simulink model "Heating_system"  (R2021a)
settings: Solver=VariableStepAuto  StartTime=0.0  StopTime=inf  RelTol=1e-3
settings Model: DataDictionary=Thermostat.sldd  EnablePacing=on  PacingRate=0.350000  OrderedModelArguments=off  Creator=smrh1  LastModifiedBy=smrh1

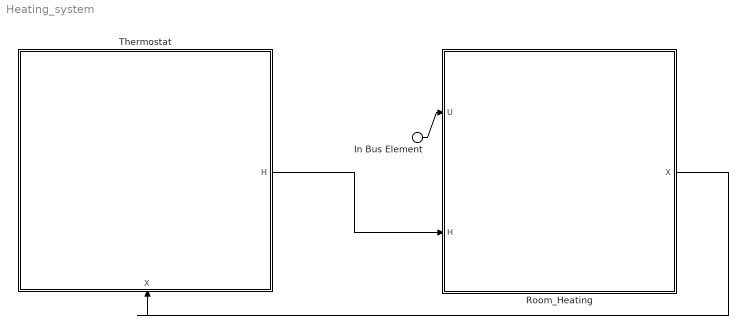
== system Heating_system ==
  In Bus Element : Inport  PortName=U
  Room_Heating : Subsystem
      settings: PortSchema="{\"entries\":[{\"content\":{\"headerSize\":26,\"margin\":15,\"minimumSpacing\":25,\"sides\":[{\"content\":{\"connectorIds\":[\"In1\",\"In2\"]},\"type\":\"ConnectorPlacement.EquallySpacedRectSide\",\"uuid\":\"3399fd0f-e173-41a6-b187-8436c8bfa551\"},{\"content\":{\"connectorIds\":[\"Out1\"],\"side\":\"RIGHT\"},\"type\":\"ConnectorPlacement.EquallySpacedRectSide\",\"uuid\":\"ade3010a-e700-4d19-9692-9b4fbd9f77bd\"},{\"content\":{\"connectorIds\":[],\"side\":\"TOP\"},\"type\":\"ConnectorPlacement.EquallySpacedRectSide\",\"uuid\":\"996f7f95-9ab9-4e94-926a-d72fb20bb1ec\"}]},\"type\":\"ConnectorPlacement.EquallySpacedConnector\",\"uuid\":\"0c58a4e7-12d7-4b31-b33f-6c78252624a7\"}],\"packageUris\":[\"http://schema.mathworks.com/mf0/Connector/R2020b\"],\"version\":\"1.0\"}"
  Thermostat : Subsystem
      settings: PortSchema="{\"entries\":[{\"content\":{\"headerSize\":26,\"margin\":15,\"minimumSpacing\":25,\"sides\":[{\"content\":{\"connectorIds\":[]},\"type\":\"ConnectorPlacement.EquallySpacedRectSide\",\"uuid\":\"3399fd0f-e173-41a6-b187-8436c8bfa551\"},{\"content\":{\"connectorIds\":[\"Out1\"],\"side\":\"RIGHT\"},\"type\":\"ConnectorPlacement.EquallySpacedRectSide\",\"uuid\":\"ade3010a-e700-4d19-9692-9b4fbd9f77bd\"},{\"content\":{\"connectorIds\":[],\"side\":\"TOP\"},\"type\":\"ConnectorPlacement.EquallySpacedRectSide\",\"uuid\":\"996f7f95-9ab9-4e94-926a-d72fb20bb1ec\"},{\"content\":{\"connectorIds\":[\"In1\"],\"side\":\"BOTTOM\"},\"type\":\"ConnectorPlacement.EquallySpacedRectSide\",\"uuid\":\"850434b0-8785-4975-a631-b4ec0ca1fe29\"}]},\"type\":\"ConnectorPlacement.EquallySpacedConnector\",\"uuid\":\"0c58a4e7-12d7-4b31-b33f-6c78252624a7\"}],\"packageUris\":[\"http://schema.mathworks.com/mf0/Connector/R2020b\"],\"version\":\"1.0\"}"
  wires:
  Thermostat/1(H) -> Room_Heating/2(H)
  In Bus Element/1 -> Room_Heating/1(U)
  Room_Heating/1(X) -> Thermostat/1(X)

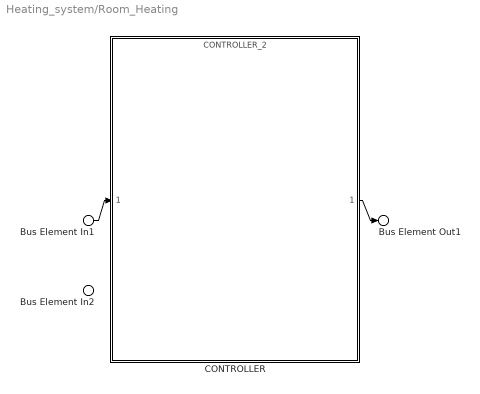
== system Heating_system/Room_Heating ==
  Bus Element In2 : Inport  PortName=U
  Bus Element In1 : Inport  Port=2  PortName=H
  CONTROLLER : ModelReference  ModelNameDialog=CONTROLLER_2  SimulationMode=Normal  ModelReferenceVersion=1.8
      settings: PortSchema="{\"entries\":[{\"content\":{\"headerSize\":38,\"margin\":15,\"minimumSpacing\":25,\"sides\":[{\"content\":{\"connectorIds\":[\"In1\"]},\"type\":\"ConnectorPlacement.EquallySpacedRectSide\",\"uuid\":\"3b44bb81-377b-4962-9dcc-156f7f1f6855\"},{\"content\":{\"connectorIds\":[\"Out1\"],\"side\":\"RIGHT\"},\"type\":\"ConnectorPlacement.EquallySpacedRectSide\",\"uuid\":\"4cba6eea-a5d9-4e03-afc9-ce5179a534ee\"},{\"content\":{\"connectorIds\":[],\"side\":\"TOP\"},\"type\":\"ConnectorPlacement.EquallySpacedRectSide\",\"uuid\":\"ada12532-fc1a-481d-80e3-afcc666e3a52\"}]},\"type\":\"ConnectorPlacement.EquallySpacedConnector\",\"uuid\":\"a760b321-2586-4ca9-a211-69f54ba7565a\"}],\"packageUris\":[\"http://schema.mathworks.com/mf0/Connector/R2020b\"],\"version\":\"1.0\"}"
  Bus Element Out1 : Outport  PortName=X
  wires:
  Bus Element In1/1 -> CONTROLLER/1
  CONTROLLER/1 -> Bus Element Out1/1

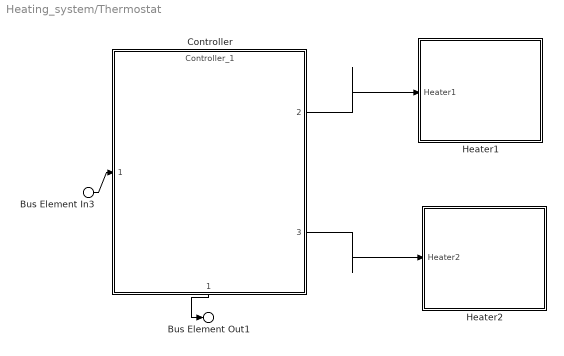
== system Heating_system/Thermostat ==
  Bus Element In3 : Inport  PortName=X
  Controller : ModelReference  ModelNameDialog=Controller_1  SimulationMode=Normal  ModelReferenceVersion=1.14
      settings: PortSchema="{\"entries\":[{\"content\":{\"headerSize\":38,\"margin\":15,\"minimumSpacing\":25,\"sides\":[{\"content\":{\"connectorIds\":[\"In1\"]},\"type\":\"ConnectorPlacement.EquallySpacedRectSide\",\"uuid\":\"3b44bb81-377b-4962-9dcc-156f7f1f6855\"},{\"content\":{\"connectorIds\":[\"Out2\",\"Out3\"],\"side\":\"RIGHT\"},\"type\":\"ConnectorPlacement.EquallySpacedRectSide\",\"uuid\":\"4cba6eea-a5d9-4e03-afc9-ce5179a534ee\"},{\"content\":{\"connectorIds\":[],\"side\":\"TOP\"},\"type\":\"ConnectorPlacement.EquallySpacedRectSide\",\"uuid\":\"ada12532-fc1a-481d-80e3-afcc666e3a52\"},{\"content\":{\"connectorIds\":[\"Out1\"],\"side\":\"BOTTOM\"},\"type\":\"ConnectorPlacement.EquallySpacedRectSide\",\"uuid\":\"294716b9-12bb-4ef2-b724-e28be1042d03\"}]},\"type\":\"ConnectorPlacement.EquallySpacedConnector\",\"uuid\":\"a760b321-2586-4ca9-a211-69f54ba7565a\"}],\"packageUris\":[\"http://schema.mathworks.com/mf0/Connector/R2020b\"],\"version\":\"1.0\"}"
  Heater1 : Subsystem
      settings: PortSchema="{\"entries\":[{\"content\":{\"headerSize\":26,\"margin\":15,\"minimumSpacing\":25,\"sides\":[{\"content\":{\"connectorIds\":[\"In1\"]},\"type\":\"ConnectorPlacement.EquallySpacedRectSide\",\"uuid\":\"3b44bb81-377b-4962-9dcc-156f7f1f6855\"},{\"content\":{\"connectorIds\":[],\"side\":\"RIGHT\"},\"type\":\"ConnectorPlacement.EquallySpacedRectSide\",\"uuid\":\"4cba6eea-a5d9-4e03-afc9-ce5179a534ee\"},{\"content\":{\"connectorIds\":[],\"side\":\"TOP\"},\"type\":\"ConnectorPlacement.EquallySpacedRectSide\",\"uuid\":\"ada12532-fc1a-481d-80e3-afcc666e3a52\"}]},\"type\":\"ConnectorPlacement.EquallySpacedConnector\",\"uuid\":\"a760b321-2586-4ca9-a211-69f54ba7565a\"}],\"packageUris\":[\"http://schema.mathworks.com/mf0/Connector/R2020b\"],\"version\":\"1.0\"}"
  Heater2 : Subsystem
      settings: PortSchema="{\"entries\":[{\"content\":{\"headerSize\":26,\"margin\":15,\"minimumSpacing\":25,\"sides\":[{\"content\":{\"connectorIds\":[\"In1\"]},\"type\":\"ConnectorPlacement.EquallySpacedRectSide\",\"uuid\":\"3b44bb81-377b-4962-9dcc-156f7f1f6855\"},{\"content\":{\"connectorIds\":[],\"side\":\"RIGHT\"},\"type\":\"ConnectorPlacement.EquallySpacedRectSide\",\"uuid\":\"4cba6eea-a5d9-4e03-afc9-ce5179a534ee\"},{\"content\":{\"connectorIds\":[],\"side\":\"TOP\"},\"type\":\"ConnectorPlacement.EquallySpacedRectSide\",\"uuid\":\"ada12532-fc1a-481d-80e3-afcc666e3a52\"}]},\"type\":\"ConnectorPlacement.EquallySpacedConnector\",\"uuid\":\"a760b321-2586-4ca9-a211-69f54ba7565a\"}],\"packageUris\":[\"http://schema.mathworks.com/mf0/Connector/R2020b\"],\"version\":\"1.0\"}"
  Bus Element Out1 : Outport  PortName=H
  wires:
  Controller/1 -> Bus Element Out1/1
  Controller/2 -> Heater1/1(Heater1)
  Controller/3 -> Heater2/1(Heater2)
  Bus Element In3/1 -> Controller/1

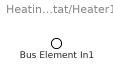
== system Heating_system/Thermostat/Heater1 ==
  Bus Element In1 : Inport  PortName=Heater1

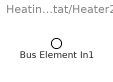
== system Heating_system/Thermostat/Heater2 ==
  Bus Element In1 : Inport  PortName=Heater2
